simulink model "observer"  (R2022b)
settings: Solver=VariableStepAuto  StartTime=0.0  StopTime=200  RelTol=1e-3
undefined symbols (not defined in the file): A, B, C, d1, d2, DZ, I, km, L, MAX_PWM, miu, SysHat, wb, wcp, wm
settings Model: Creator=amoralesma  LastModifiedBy=felip

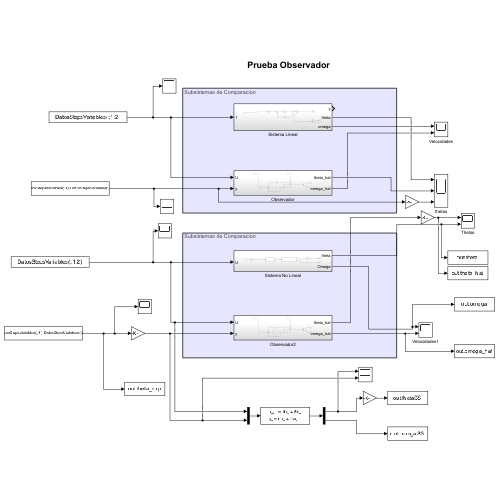
[thumbnail: Simulink's stored preview of the top-level diagram]
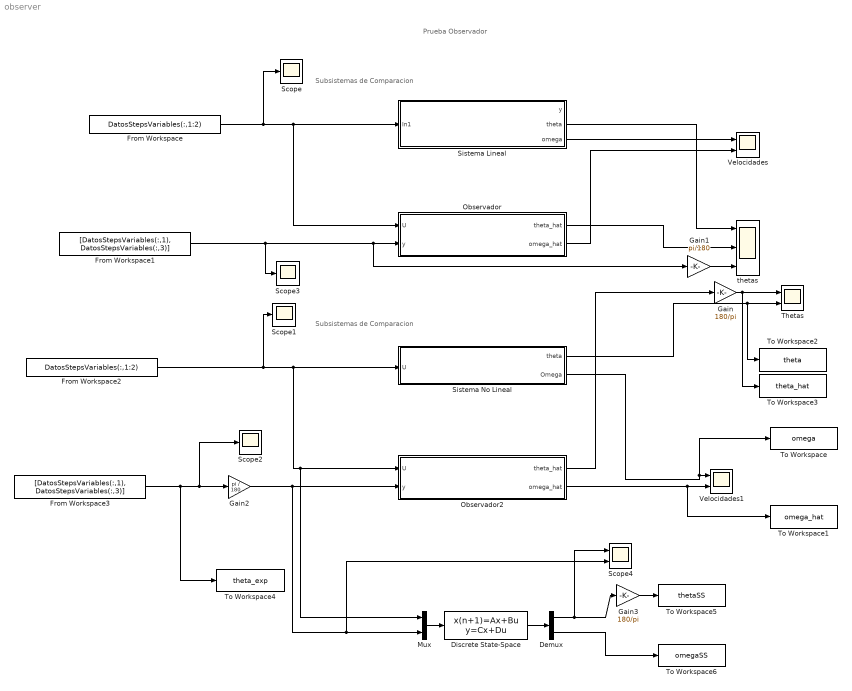
== system observer ==
  note: Subsistemas de Comparacion
  note: Prueba Observador
  note: Subsistemas de Comparacion
  Demux : Demux  Outputs=2
  Discrete State-Space : DiscreteStateSpace  A=SysHat.A  B=SysHat.B  C=SysHat.C  D=SysHat.D  SampleTime=2.5e-3
  From Workspace : FromWorkspace  VariableName=DatosStepsVariables(:,1:2)  SampleTime=2.5e-3
  From Workspace1 : FromWorkspace  VariableName=[DatosStepsVariables(:,1), DatosStepsVariables(:,3)]  SampleTime=2.5e-3
  From Workspace2 : FromWorkspace  VariableName=DatosStepsVariables(:,1:2)  SampleTime=2.5e-3
  From Workspace3 : FromWorkspace  VariableName=[DatosStepsVariables(:,1), DatosStepsVariables(:,3)]  SampleTime=2.5e-3
  Gain : Gain  Gain=180/pi
  Gain1 : Gain  Gain=pi/180
  Gain2 : Gain  Gain=pi / 180
  Gain3 : Gain  Gain=180/pi
  Mux : Mux  Inputs=2
  Observador : Subsystem
  Observador2 : Subsystem
  Scope{,1..3} (4 alike) : Scope
  Scope4 : Scope  NumInputPorts=2
  Sistema Lineal : Subsystem
  Sistema No Lineal : Subsystem
  Thetas : Scope  NumInputPorts=2
  To Workspace : ToWorkspace  VariableName=omega  SaveFormat=Timeseries  SampleTime=-1
  To Workspace1 : ToWorkspace  VariableName=omega_hat  SaveFormat=Timeseries  SampleTime=-1
  To Workspace2 : ToWorkspace  VariableName=theta  SaveFormat=Timeseries  SampleTime=-1
  To Workspace3 : ToWorkspace  VariableName=theta_hat  SaveFormat=Timeseries  SampleTime=-1
  To Workspace4 : ToWorkspace  VariableName=theta_exp  SaveFormat=Timeseries  SampleTime=-1
  To Workspace5 : ToWorkspace  VariableName=thetaSS  SaveFormat=Timeseries  SampleTime=-1
  To Workspace6 : ToWorkspace  VariableName=omegaSS  SaveFormat=Timeseries  SampleTime=-1
  Velocidades : Scope  NumInputPorts=2
  Velocidades1 : Scope  NumInputPorts=2
  thetas : Scope  NumInputPorts=3
  wires:
  From Workspace/1 -> Observador/1(U), Sistema Lineal/1(In1), Scope/1
  From Workspace1/1 -> Scope3/1, Gain1/1, Observador/2(y)
  Sistema Lineal/3(omega) -> Velocidades/1
  Observador/2(omega_hat) -> Velocidades/2
  Sistema No Lineal/2(Omega) -> To Workspace/1, Velocidades1/1
  From Workspace2/1 -> Scope1/1, Sistema No Lineal/1(U), Mux/1, Observador2/1(U)
  From Workspace3/1 -> Scope2/1, Gain2/1, To Workspace4/1
  Observador2/2(omega_hat) -> Velocidades1/2, To Workspace1/1
  Sistema No Lineal/1(theta) -> To Workspace2/1, Thetas/2
  Observador2/1(theta_hat) -> Gain/1
  Gain/1 -> To Workspace3/1, Thetas/1
  Observador/1(theta_hat) -> thetas/2
  Sistema Lineal/2(theta) -> thetas/1
  Gain1/1 -> thetas/3
  Gain2/1 -> Scope4/2, Mux/2, Observador2/2(y)
  Demux/1 -> Scope4/1, Gain3/1
  Demux/2 -> To Workspace6/1
  Gain3/1 -> To Workspace5/1
  Mux/1 -> Discrete State-Space/1
  Discrete State-Space/1 -> Demux/1

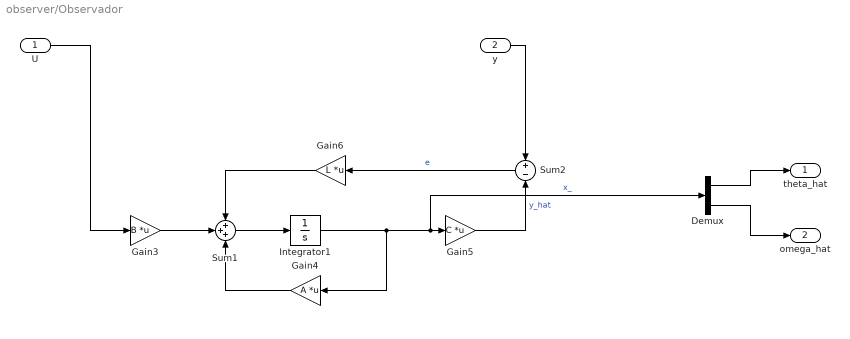
== system observer/Observador ==
  U : Inport
  y : Inport  Port=2
  Demux : Demux  Outputs=2
  Gain3 : Gain  Gain=B  Multiplication=Matrix(K*u)
  Gain4 : Gain  Gain=A  Multiplication=Matrix(K*u)
  Gain5 : Gain  Gain=C  Multiplication=Matrix(K*u)
  Gain6 : Gain  Gain=L  Multiplication=Matrix(K*u)
  Integrator1 : Integrator
  Sum1 : Sum  Inputs=+++
  Sum2 : Sum  Inputs=+|-
  theta_hat : Outport
  omega_hat : Outport  Port=2
  wires:
  U/1 -> Gain3/1
  y/1 -> Sum2/1
  Gain5/1 -> Sum2/2  "y_hat"
  Sum1/1 -> Integrator1/1
  Gain3/1 -> Sum1/2
  Gain6/1 -> Sum1/1
  Integrator1/1 -> Gain4/1, Demux/1, Gain5/1  "x_"
  Sum2/1 -> Gain6/1  "e"
  Gain4/1 -> Sum1/3
  Demux/1 -> theta_hat/1
  Demux/2 -> omega_hat/1

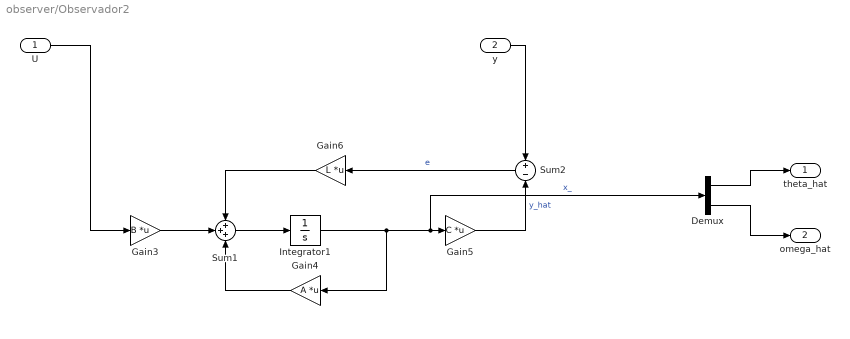
== system observer/Observador2 ==
  U : Inport
  y : Inport  Port=2
  Demux : Demux  Outputs=2
  Gain3 : Gain  Gain=B  Multiplication=Matrix(K*u)
  Gain4 : Gain  Gain=A  Multiplication=Matrix(K*u)
  Gain5 : Gain  Gain=C  Multiplication=Matrix(K*u)
  Gain6 : Gain  Gain=L  Multiplication=Matrix(K*u)
  Integrator1 : Integrator  InitialCondition=[deg2rad(10), 0]
  Sum1 : Sum  Inputs=+++
  Sum2 : Sum  Inputs=+|-
  theta_hat : Outport
  omega_hat : Outport  Port=2
  wires:
  U/1 -> Gain3/1
  y/1 -> Sum2/1
  Gain5/1 -> Sum2/2  "y_hat"
  Sum1/1 -> Integrator1/1
  Gain3/1 -> Sum1/2
  Gain6/1 -> Sum1/1
  Integrator1/1 -> Gain4/1, Demux/1, Gain5/1  "x_"
  Sum2/1 -> Gain6/1  "e"
  Gain4/1 -> Sum1/3
  Demux/1 -> theta_hat/1
  Demux/2 -> omega_hat/1

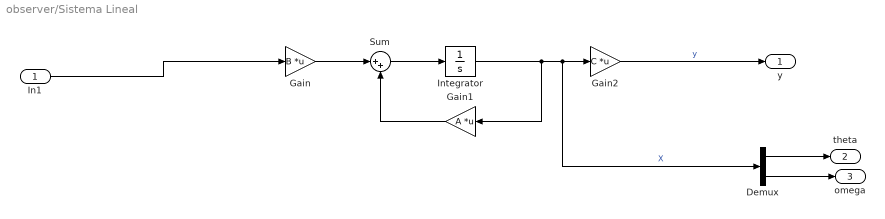
== system observer/Sistema Lineal ==
  In1 : Inport
  Demux : Demux  Outputs=2
  Gain : Gain  Gain=B  Multiplication=Matrix(K*u)
  Gain1 : Gain  Gain=A  Multiplication=Matrix(K*u)
  Gain2 : Gain  Gain=C  Multiplication=Matrix(K*u)
  Integrator : Integrator
  Sum : Sum  Inputs=|++
  y : Outport
  theta : Outport  Port=2
  omega : Outport  Port=3
  wires:
  In1/1 -> Gain/1
  Gain1/1 -> Sum/2
  Sum/1 -> Integrator/1
  Integrator/1 -> Gain1/1, Demux/1, Gain2/1  "X"
  Gain2/1 -> y/1  "y"
  Gain/1 -> Sum/1
  Demux/1 -> theta/1
  Demux/2 -> omega/1

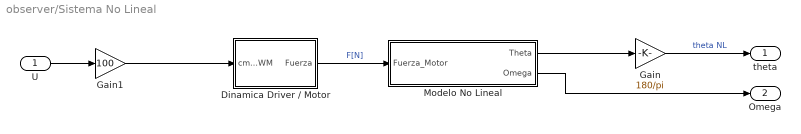
== system observer/Sistema No Lineal ==
  U : Inport
  Dinamica Driver / Motor : Subsystem
  Gain : Gain  Gain=180/pi
  Gain1 : Gain  Gain=100
  Modelo No Lineal : Subsystem
  theta : Outport
  Omega : Outport  Port=2
  wires:
  Gain/1 -> theta/1  "theta NL"
  Modelo No Lineal/1(Theta) -> Gain/1
  Modelo No Lineal/2(Omega) -> Omega/1
  Dinamica Driver / Motor/1(Fuerza) -> Modelo No Lineal/1(Fuerza_Motor)  "F[N]"
  Gain1/1 -> Dinamica Driver / Motor/1(cmd_PWM)
  U/1 -> Gain1/1

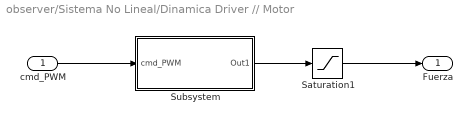
== system observer/Sistema No Lineal/Dinamica Driver // Motor ==
  cmd_PWM : Inport
  Saturation1 : Saturate  UpperLimit=MAX_PWM
  Subsystem : Subsystem
  Fuerza : Outport
  wires:
  Saturation1/1 -> Fuerza/1
  cmd_PWM/1 -> Subsystem/1(cmd_PWM)
  Subsystem/1(Out1) -> Saturation1/1

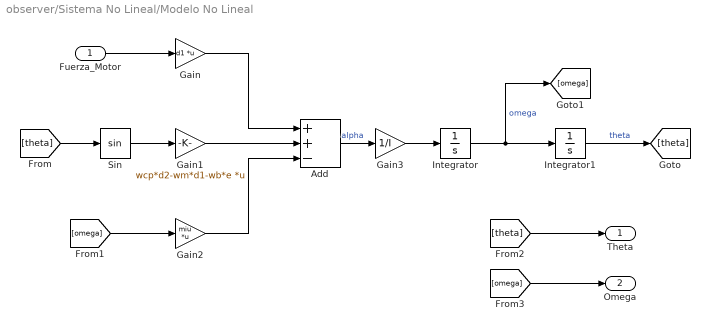
== system observer/Sistema No Lineal/Modelo No Lineal ==
  Fuerza_Motor : Inport
  Add : Sum  Inputs=++-
  Gain : Gain  Gain=d1  Multiplication=Matrix(K*u)
  Gain1 : Gain  Gain=wcp*d2-wm*d1-wb*e  Multiplication=Matrix(K*u)
  Gain2 : Gain  Gain=miu  Multiplication=Matrix(K*u)
  Gain3 : Gain  Gain=1/I
  Integrator : Integrator
  Integrator1 : Integrator
  Sin : Trigonometry
  Theta : Outport
  Omega : Outport  Port=2
  wires:
  [omega] -> Omega/1
  Gain1/1 -> Add/2
  Integrator/1 -> [omega], Integrator1/1  "omega"
  Fuerza_Motor/1 -> Gain/1
  Integrator1/1 -> [theta]  "theta"
  Gain2/1 -> Add/3
  Gain/1 -> Add/1
  Add/1 -> Gain3/1  "alpha"
  [theta] -> Sin/1
  [omega] -> Gain2/1
  [theta] -> Theta/1
  Sin/1 -> Gain1/1
  Gain3/1 -> Integrator/1

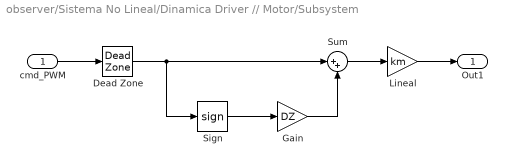
== system observer/Sistema No Lineal/Dinamica Driver // Motor/Subsystem ==
  cmd_PWM : Inport
  Dead Zone : DeadZone  LowerValue=-DZ  UpperValue=DZ
  Gain : Gain  Gain=DZ
  Lineal : Gain  Gain=km
  Sign : Signum
  Sum : Sum  Inputs=|++
  Out1 : Outport
  wires:
  cmd_PWM/1 -> Dead Zone/1
  Dead Zone/1 -> Sum/1, Sign/1
  Sum/1 -> Lineal/1
  Sign/1 -> Gain/1
  Gain/1 -> Sum/2
  Lineal/1 -> Out1/1
